simulink model "DCMotor_PIDControl"  (R2021b)
settings: Solver=VariableStepAuto  StartTime=0.0  StopTime=10  RelTol=1e-3
InitFcn:
  | dcMotorParams
values from neighbouring files (symbols this model uses):
  b = 0.1    [dcMotorParams.m]
  J = 0.01    [dcMotorParams.m]
  K_EMF = 0.01    [dcMotorParams.m]
  K_T = 0.01    [dcMotorParams.m]
  L = 0.5    [dcMotorParams.m]
  R = 1    [dcMotorParams.m]
libraries: simulink x1, slpidlib x1
settings Model: Creator=ecosg  LastModifiedBy=ecosg

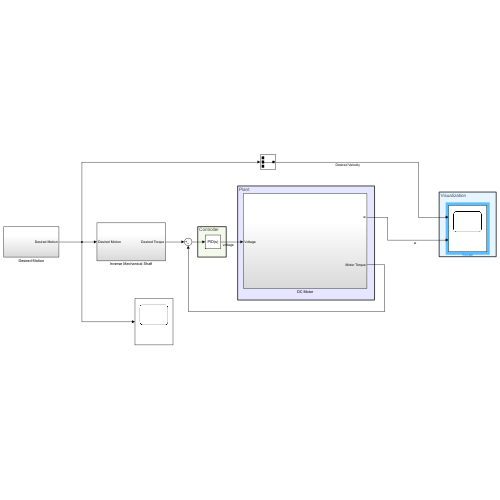
[thumbnail: Simulink's stored preview of the top-level diagram]
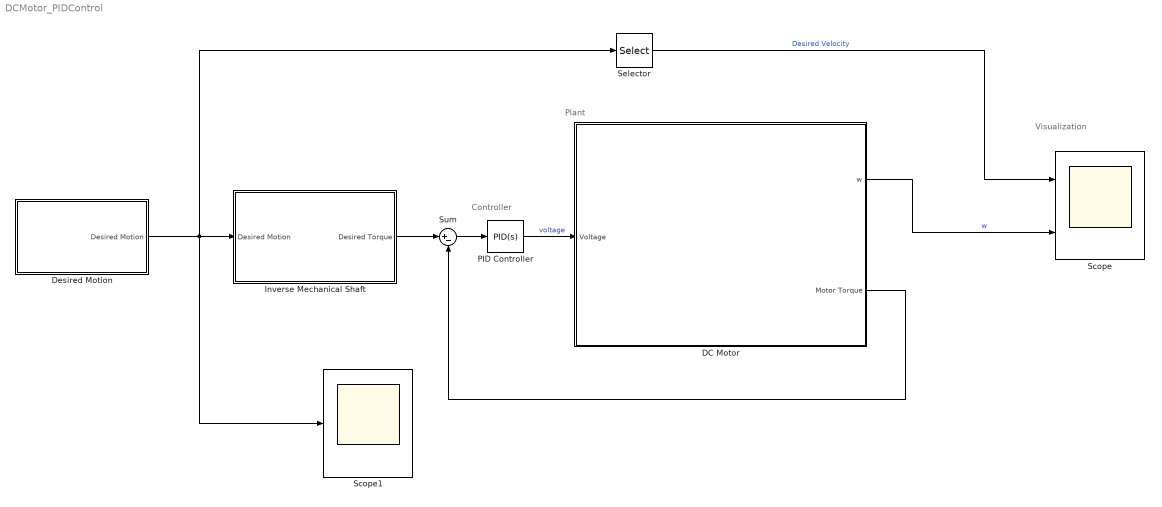
== system DCMotor_PIDControl ==
  note: Controller
  note: Plant
  note: Visualization
  DC Motor : Subsystem
  Desired Motion : Subsystem
  Inverse Mechanical Shaft : Subsystem
  PID Controller : slpidlib/PID Controller  Controller=PID  Form=Parallel  TimeDomain=Continuous-time  UseExternalTs=off  SampleTime=-1  IntegratorMethod=Forward Euler  FilterMethod=Forward Euler  ControllerParametersSource=internal  P=1  I=1  D=0  UseFilter=on  N=1  TunerSelectOption=Transfer Function Based (PID Tuner App)  InitialConditionSource=internal  InitialConditionForIntegrator=0  InitialConditionForFilter=0  DifferentiatorICPrevScaledInput=0  ExternalReset=none  TrackingMode=off  Kt=1  LimitOutput=off  SatLimitsSource=internal  UpperSaturationLimit=inf  LowerSaturationLimit=-inf  LinearizeAsGain=on  AntiWindupMode=none  Kb=1  POutMin=[]  POutMax=[]  IOutMin=[]  IOutMax=[]  DOutMin=[]  DOutMax=[]  NOutMin=[]  NOutMax=[]  SumOutMin=[]  SumOutMax=[]  SaturationOutMin=[]  SaturationOutMax=[]  PParamMin=[]  PParamMax=[]  IParamMin=[]  IParamMax=[]  DParamMin=[]  DParamMax=[]  NParamMin=[]  NParamMax=[]  KbParamMin=[]  KbParamMax=[]  KtParamMin=[]  KtParamMax=[]  KbOutMin=[]  KbOutMax=[]  KtOutMin=[]  KtOutMax=[]  IntegratorOutMin=[]  IntegratorOutMax=[]  FilterOutMin=[]  FilterOutMax=[]  SumI1OutMin=[]  SumI1OutMax=[]  SumI2OutMin=[]  SumI2OutMax=[]  SumI3OutMin=[]  SumI3OutMax=[]  SumI4OutMin=[]  SumI4OutMax=[]  SumDOutMin=[]  SumDOutMax=[]  DifferentiatorOutMin=[]  DifferentiatorOutMax=[]  FilterDiffOutCoefMin=[]  FilterDiffOutCoefMax=[]  ReciprocalOutMin=[]  ReciprocalOutMax=[]  SumDenOutMin=[]  SumDenOutMax=[]  SumNumOutMin=[]  SumNumOutMax=[]  DivideOutMin=[]  DivideOutMax=[]  UdiffTsProdOutMin=[]  UdiffTsProdOutMax=[]  NTsProdOutMin=[]  NTsProdOutMax=[]  UintegralTsProdOutMin=[]  UintegralTsProdOutMax=[]  UngainTsProdOutMin=[]  UngainTsProdOutMax=[]  IntegratorContinuousStateAttributes=''  IntegratorStateMustResolveToSignalObject=off  IntegratorRTWStateStorageClass=Auto  FilterContinuousStateAttributes=''  FilterStateMustResolveToSignalObject=off  FilterRTWStateStorageClass=Auto  ParallelPVariant=InternalParameters  IdealPVariant=Disabled  IVariant=InternalParameters  DVariant=InternalParameters  IntegratorVariant=Continuous  SatVariant=Disabled  AWVariant=Passthrough  PCopyVariant=Disabled  TRVariant=Disabled  FdbkBlocksVariant=Forward  IdealPFdbkVariant=Disabled  SatFdbkVariant=Disabled  DerivativeFilterVariant=ContFilter  NVariant=InternalParameters  NCopyVariant=Disabled  FilterICVariant=InternalICsFilter  IntegratorICVariant=InternalICs  ExternalResetVariant=Disabled  TRSumVariant=Passthrough  SumFdbkVariant=Disabled  SumVariant=Sum_PID  TsampFilterVariant=InternalTs  TsampNgainVariant=Passthrough  TsampIntegralVariant=Passthrough  ExternalSaturationOutDataTypeStr=Inherit: Same as second input
  Scope : Scope  NumInputPorts=2
  Scope1 : Scope
  Selector : Selector  InputPortWidth=3  IndexOptions=Index vector (dialog)  Indices=2  OutputSizes=1
  Sum : Sum  Inputs=|+-
  wires:
  DC Motor/1(w) -> Scope/2  "w"
  Sum/1 -> PID Controller/1
  PID Controller/1 -> DC Motor/1(Voltage)  "voltage"
  DC Motor/2(Motor Torque) -> Sum/2
  Inverse Mechanical Shaft/1(Desired Torque) -> Sum/1
  Desired Motion/1(Desired Motion) -> Scope1/1, Selector/1, Inverse Mechanical Shaft/1(Desired Motion)
  Selector/1 -> Scope/1  "Desired Velocity"

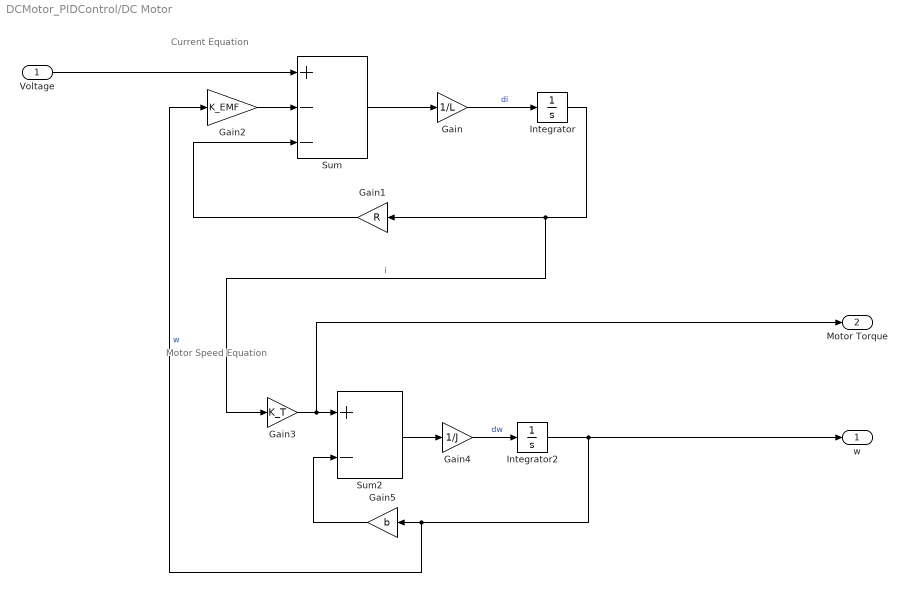
== system DCMotor_PIDControl/DC Motor ==
  note: Motor Speed Equation
  note: Current Equation
  Voltage : Inport
  Gain : Gain  Gain=1/L
  Gain1 : Gain  Gain=R
  Gain2 : Gain  Gain=K_EMF
  Gain3 : Gain  Gain=K_T
  Gain4 : Gain  Gain=1/J
  Gain5 : Gain  Gain=b
  Integrator : Integrator
  Integrator2 : Integrator
  Sum : Sum  Inputs=+--
  Sum2 : Sum  Inputs=+-
  w : Outport
  Motor Torque : Outport  Port=2
  wires:
  Integrator2/1 -> w/1, Gain2/1, Gain5/1  "w"
  Gain4/1 -> Integrator2/1  "dw"
  Gain5/1 -> Sum2/2
  Sum/1 -> Gain/1
  Integrator/1 -> Gain1/1, Gain3/1  "i"
  Sum2/1 -> Gain4/1
  Gain/1 -> Integrator/1  "di"
  Gain1/1 -> Sum/3
  Gain2/1 -> Sum/2
  Voltage/1 -> Sum/1
  Gain3/1 -> Motor Torque/1, Sum2/1

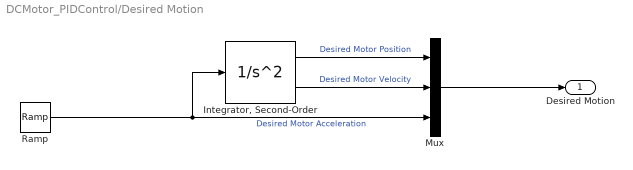
== system DCMotor_PIDControl/Desired Motion ==
  "Integrator, Second-Order" : SecondOrderIntegrator
  Mux : Mux  Inputs=3
  Ramp : simulink/Sources/Ramp  slope=-6*pi/250  start=0  InitialOutput=3*pi/25
  Desired Motion : Outport
  wires:
  Ramp/1 -> "Integrator, Second-Order"/1, Mux/3  "Desired Motor Acceleration"
  "Integrator, Second-Order"/1 -> Mux/1  "Desired Motor Position"
  "Integrator, Second-Order"/2 -> Mux/2  "Desired Motor Velocity"
  Mux/1 -> Desired Motion/1

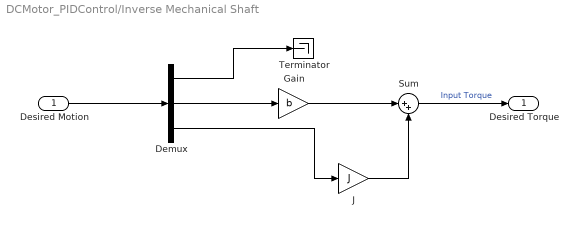
== system DCMotor_PIDControl/Inverse Mechanical Shaft ==
  Desired Motion : Inport
  Demux : Demux  Outputs=3
  Gain : Gain  Gain=b
  J : Gain  Gain=J
  Sum : Sum  Inputs=|++
  Terminator : Terminator
  Desired Torque : Outport
  wires:
  Gain/1 -> Sum/1
  J/1 -> Sum/2
  Sum/1 -> Desired Torque/1  "Input Torque"
  Desired Motion/1 -> Demux/1
  Demux/2 -> Gain/1
  Demux/3 -> J/1
  Demux/1 -> Terminator/1
